simulink model "PID"  (R2023a)
settings: Solver=VariableStepAuto  StartTime=0.0  StopTime=30.0  RelTol=1e-3
settings Model: Creator=ihsan  LastModifiedBy=ihsan

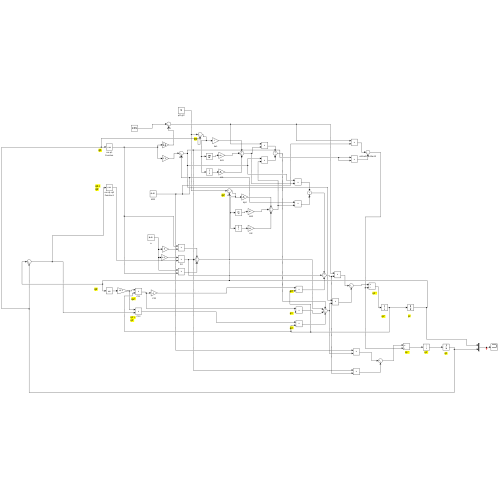
[thumbnail: Simulink's stored preview of the top-level diagram]
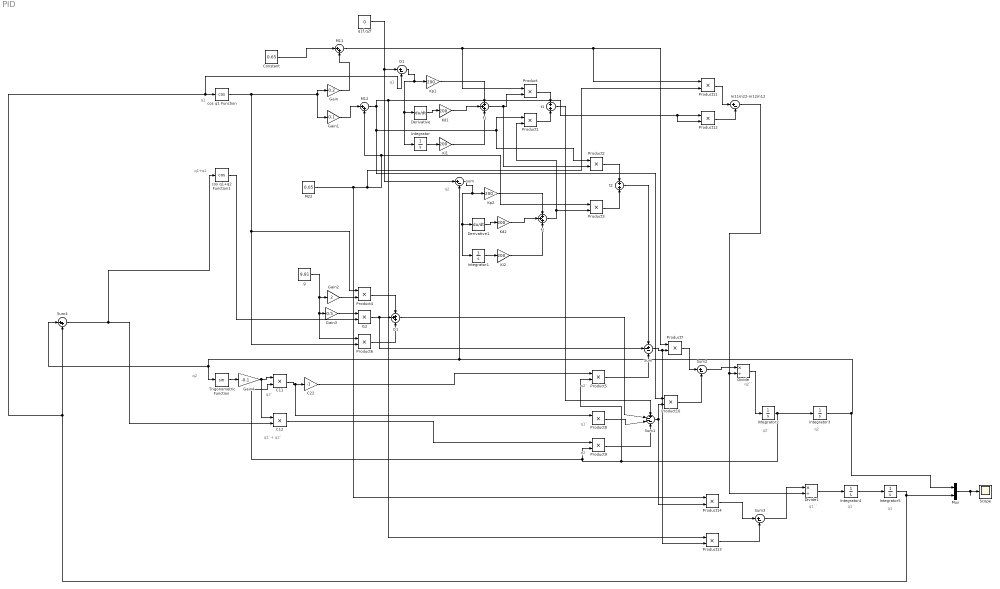
== system PID ==
  note: q1
  note: q1`
  note: q1``
  note: q2
  note: q2`
  note: q2``
  note: q2`
  note: q1`
  note: q2`
  note: q1`+
      | q2`
  note: q1
  note: q1
  note: q1+q2
  note: q2
  note: q2`
  note: q2
  C11 : Product
  C12 : Product
  C22 : Gain  Gain=-1
  Constant : Constant  Value=0.65
  Derivative : Derivative
  Derivative1 : Derivative
  Divide : Product  Inputs=*/
  Divide1 : Product  Inputs=*/
  G1 : Sum  Inputs=+++
  G2 : Product
  Gain : Gain  Gain=0.2
  Gain1 : Gain  Gain=0.1
  Gain2 : Gain  Gain=2
  Gain3 : Gain  Gain=0.5
  Gain4 : Gain  Gain=-0.1
  Integrator{,1..2,4} (4 alike) : Integrator
  Integrator3 : Integrator  InitialCondition=0.1
  Integrator5 : Integrator  InitialCondition=0.1
  Kd1 : Gain  Gain=200
  Kd2 : Gain  Gain=200
  Ki1 : Gain  Gain=200
  Ki2 : Gain  Gain=200
  Kp1 : Gain  Gain=200
  Kp2 : Gain  Gain=200
  M11 : Sum  Inputs=|++
  M12 : Sum  Inputs=|++
  M22 : Constant  Value=0.05
  Mux : Mux  Inputs=2
  Product{,1..14} (15 alike) : Product
  Q1 : Sum  Inputs=|+-
  Scope : Scope
  Sum : Sum  Inputs=+--
  Sum1 : Sum  Inputs=+---
  Sum2 : Sum  Inputs=|+-
  Sum3 : Sum  Inputs=|+-
  Sum4 : Sum  Inputs=|++
  Trigonometric Function : Trigonometry
  cos q1 Function : Trigonometry  Operator=cos
  cos q1+q2 Function1 : Trigonometry  Operator=cos
  f1 : Sum  Inputs=+++
  f2 : Sum  Inputs=+++
  g : Constant  Value=9.81
  m11m22-m12m12 : Sum  Inputs=|+-
  q1f,q2f : Constant  Value=0
  sum : Sum  Inputs=|+-
  t1 : Sum
  t2 : Sum
  wires:
  cos q1 Function/1 -> Product6/2, Product4/1, Gain/1, Gain1/1
  Constant/1 -> M11/1
  Gain/1 -> M11/2
  Gain1/1 -> M12/1
  M22/1 -> Product14/1, Product11/2, Product3/1, M12/2
  q1f,q2f/1 -> Q1/1, sum/1
  Q1/1 -> Integrator/1, Derivative/1, Kp1/1
  Derivative/1 -> Kd1/1
  Integrator/1 -> Ki1/1
  Kp1/1 -> f1/1
  Kd1/1 -> f1/2
  Ki1/1 -> f1/3
  Kp2/1 -> f2/1
  Integrator1/1 -> Ki2/1
  Kd2/1 -> f2/2
  Ki2/1 -> f2/3
  sum/1 -> Integrator1/1, Derivative1/1, Kp2/1
  Derivative1/1 -> Kd2/1
  M11/1 -> Product11/1, Product7/1, Product/1
  f1/1 -> Product2/2, Product/2
  M12/1 -> Product10/1, Product2/1, Product1/1, Product13/1, Product12/2, Product12/1
  f2/1 -> Product3/2, Product1/2
  Product1/1 -> t1/2
  Product/1 -> t1/1
  Product3/1 -> t2/2
  Product2/1 -> t2/1
  g/1 -> Product6/1, Gain3/1, Gain2/1
  Gain2/1 -> Product4/2
  Gain3/1 -> G2/1
  cos q1+q2 Function1/1 -> G2/2
  Product4/1 -> G1/1
  G2/1 -> Sum/2, G1/2
  Product6/1 -> G1/3
  Trigonometric Function/1 -> Gain4/1
  Gain4/1 -> C12/1, C11/1
  C11/1 -> Product8/1, C22/1
  C22/1 -> Product5/1
  Product5/1 -> Sum/3
  t2/1 -> Sum/1
  Sum/1 -> Product13/2, Product7/2
  C12/1 -> Product9/1
  Product9/1 -> Sum1/4
  Product8/1 -> Sum1/3
  G1/1 -> Sum1/2
  t1/1 -> Sum1/1
  Sum1/1 -> Product10/2, Product14/2
  Product7/1 -> Sum2/1
  Product10/1 -> Sum2/2
  Product11/1 -> m11m22-m12m12/1
  Product12/1 -> m11m22-m12m12/2
  Sum2/1 -> Divide/1
  m11m22-m12m12/1 -> Divide1/2, Divide/2
  Divide/1 -> Integrator2/1
  Integrator2/1 -> Product5/2, C11/2, Product9/2, Integrator3/1
  Integrator3/1 -> Mux/1, Sum4/1, Trigonometric Function/1, sum/2
  Product14/1 -> Sum3/1
  Product13/1 -> Sum3/2
  Sum3/1 -> Divide1/1
  Divide1/1 -> Integrator4/1
  Integrator4/1 -> Integrator5/1
  Sum4/1 -> cos q1+q2 Function1/1, C12/2
  Integrator5/1 -> Q1/2, cos q1 Function/1, Sum4/2, Mux/2
  Mux/1 -> Scope/1
